simulink model "akshat_hwk3_p2_sim"  (R2023b)
settings: Solver=VariableStepAuto  StartTime=0.0  StopTime=25  RelTol=1e-3
values from neighbouring files (symbols this model uses):
  Kd_bar = Kd    [akshat_hwk3_p2.m]
  Ki_bar = real(Kp*PI)    [akshat_hwk3_p2.m]
  Kp_bar = real(Kp + Kd*PI)    [akshat_hwk3_p2.m]
  x_s = [pi/2; 0]    [akshat_hwk3_p2.m]
settings Model: Creator=akshatd  LastModifiedBy=akshatd

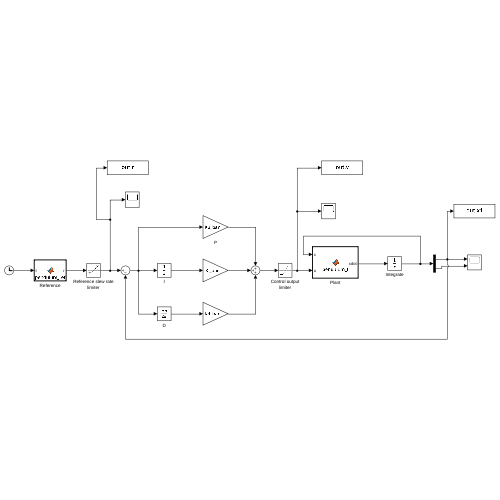
[thumbnail: Simulink's stored preview of the top-level diagram]
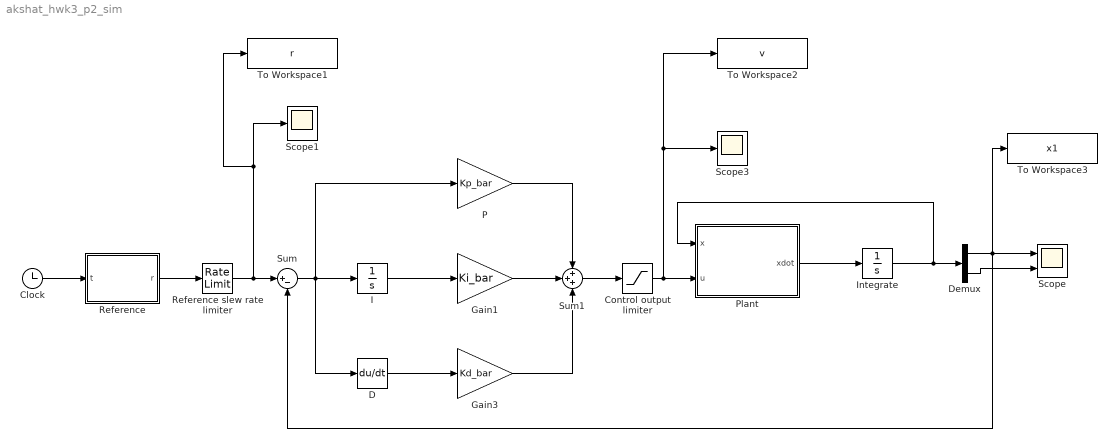
== system akshat_hwk3_p2_sim ==
  Clock : Clock
  Control output limiter : Saturate  UpperLimit=9  LowerLimit=-9
  D : Derivative
  Demux : Demux  Outputs=2
  Gain1 : Gain  Gain=Ki_bar
  Gain3 : Gain  Gain=Kd_bar
  I : Integrator
  Integrate : Integrator  InitialCondition=x_s
  P : Gain  Gain=Kp_bar
  Plant : MATLAB Function  TreatAsAtomicUnit=on
  Reference : MATLAB Function  TreatAsAtomicUnit=on
  Reference slew rate limiter : RateLimiter  RisingSlewLimit=10  FallingSlewLimit=-10  SampleTimeMode=inherited
  Scope : Scope  NumInputPorts=2
  Scope1 : Scope
  Scope3 : Scope
  Sum : Sum  Inputs=|+-
  Sum1 : Sum  Inputs=+++
  To Workspace1 : ToWorkspace  VariableName=r  SaveFormat=Timeseries  SampleTime=-1
  To Workspace2 : ToWorkspace  VariableName=v  SaveFormat=Timeseries  SampleTime=-1
  To Workspace3 : ToWorkspace  VariableName=x1  SaveFormat=Timeseries  SampleTime=-1
  wires:
  D/1 -> Gain3/1
  I/1 -> Gain1/1
  Sum1/1 -> Control output limiter/1
  Gain3/1 -> Sum1/3
  P/1 -> Sum1/1
  Sum/1 -> D/1, P/1, I/1
  Plant/1(xdot) -> Integrate/1
  Integrate/1 -> Demux/1, Plant/1(x)
  Demux/1 -> To Workspace3/1, Sum/2, Scope/1
  Demux/2 -> Scope/2
  Control output limiter/1 -> To Workspace2/1, Scope3/1, Plant/2(u)
  Clock/1 -> Reference/1(t)
  Reference/1(r) -> Reference slew rate limiter/1
  Reference slew rate limiter/1 -> To Workspace1/1, Scope1/1, Sum/1
  Gain1/1 -> Sum1/2

== matlab function akshat_hwk3_p2_sim/Plant ==
  data: x input; u input; xdot output size=2
function xdot = pendulum_f(x, u)
% x = [theta, theta_dot]
% u = [V]
% system parameters
Rm = 3.5; % Ohms, Armature resistance
Kb = 0.1; % Vs/rad, Motor back EMF constant
Kt = 0.65*Kb; % Nm/A, Motor torque constant
% Lm;  H, Armature inductance; assume 0
mp = 0.04;% kg, Spotlight(pendulum) mass
Lp = 0.1; %m, Spotlight(pendulum) length
Ip = mp*(Lp)^2;% Moment of inertia of pendulum about center of mass
Bm = 0.000008; %Nms/rad (viscous friction coefficient)
g = 9.81; %m/s^2 acceleration due to gravity

x1_dot = x(2);
x2_dot = Kt*u/(Ip*Rm) - (Kt*Kb/Rm + Bm)*x(2)/Ip - mp*g*Lp*cos(x(1))/Ip;
xdot = [x1_dot; x2_dot];
end

== matlab function akshat_hwk3_p2_sim/Reference ==
  data: t input; r output
function r = pendulum_ref(t)
if t < 5
	r = pi/2;
elseif t < 10
	r = 0;
elseif t < 15
	r = pi/2;
elseif t < 20
	r = 0;
else
	r = pi/2;
end
end
